simulink model "threephasestator"  (R2016a)
settings: Solver=VariableStepAuto  StartTime=0.0  StopTime=10.0  RelTol=1e-3
undefined symbols (not defined in the file): Lph, Rph
settings Model: Creator=rtw141  LastModifiedBy=rtw141
settings GRTTargetCC: GeneratePreprocessorConditionals=Use local settings

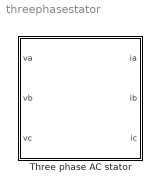
== system threephasestator ==
  Three phase AC stator : Subsystem

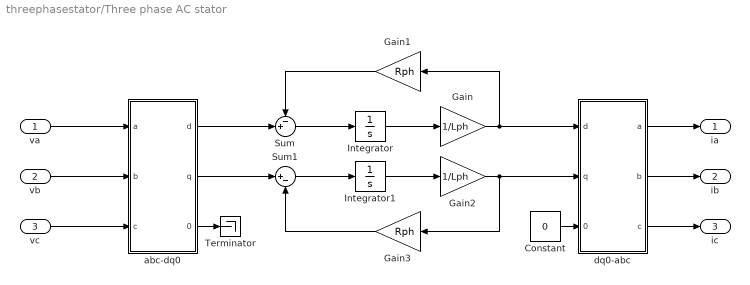
== system threephasestator/Three phase AC stator ==
  va : Inport
  vb : Inport  Port=2
  vc : Inport  Port=3
  Constant : Constant  Value=0
  Gain : Gain  Gain=1/Lph
  Gain1 : Gain  Gain=Rph
  Gain2 : Gain  Gain=1/Lph
  Gain3 : Gain  Gain=Rph
  Integrator : Integrator
  Integrator1 : Integrator
  Sum : Sum  Inputs=-+|
  Sum1 : Sum  Inputs=|+-
  Terminator : Terminator
  abc-dq0 : Subsystem
  dq0-abc : Subsystem
  ia : Outport
  ib : Outport  Port=2
  ic : Outport  Port=3
  wires:
  vc/1 -> abc-dq0/3(c)
  abc-dq0/3(0) -> Terminator/1
  va/1 -> abc-dq0/1(a)
  vb/1 -> abc-dq0/2(b)
  Gain3/1 -> Sum1/2
  Integrator/1 -> Gain/1
  dq0-abc/3(c) -> ic/1
  Sum/1 -> Integrator/1
  Gain2/1 -> dq0-abc/2(q), Gain3/1
  Gain1/1 -> Sum/1
  dq0-abc/1(a) -> ia/1
  abc-dq0/1(d) -> Sum/2
  Sum1/1 -> Integrator1/1
  Integrator1/1 -> Gain2/1
  Gain/1 -> dq0-abc/1(d), Gain1/1
  abc-dq0/2(q) -> Sum1/1
  dq0-abc/2(b) -> ib/1
  Constant/1 -> dq0-abc/3(0)

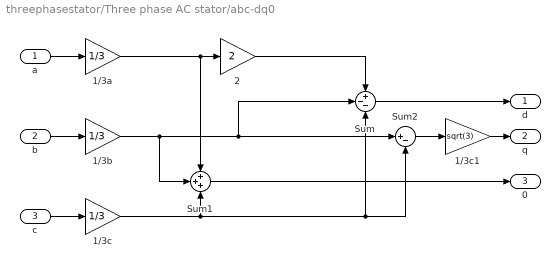
== system threephasestator/Three phase AC stator/abc-dq0 ==
  a : Inport
  b : Inport  Port=2
  c : Inport  Port=3
  1/3a : Gain  Gain=1/3
  1/3b : Gain  Gain=1/3
  1/3c : Gain  Gain=1/3
  1/3c1 : Gain  Gain=sqrt(3)
  2 : Gain  Gain=2
  Sum : Sum  Inputs=+--
  Sum1 : Sum  Inputs=+++
  Sum2 : Sum  Inputs=|+-
  d : Outport
  q : Outport  Port=2
  0 : Outport  Port=3
  wires:
  c/1 -> 1/3c/1
  b/1 -> 1/3b/1
  a/1 -> 1/3a/1
  1/3a/1 -> Sum1/1, 2/1
  2/1 -> Sum/1
  1/3b/1 -> Sum1/2, Sum2/1, Sum/2
  Sum/1 -> d/1
  1/3c/1 -> Sum1/3, Sum2/2, Sum/3
  Sum1/1 -> 0/1
  Sum2/1 -> 1/3c1/1
  1/3c1/1 -> q/1

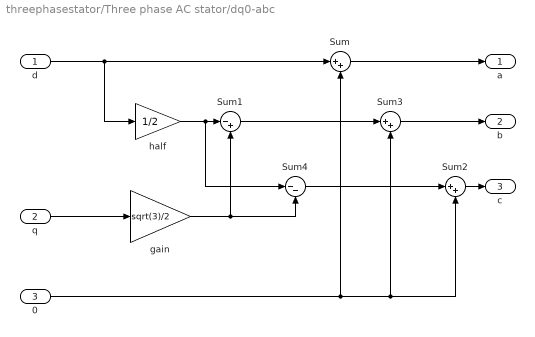
== system threephasestator/Three phase AC stator/dq0-abc ==
  d : Inport
  q : Inport  Port=2
  0 : Inport  Port=3
  Sum : Sum  Inputs=|++
  Sum1 : Sum  Inputs=|-+
  Sum2 : Sum  Inputs=|++
  Sum3 : Sum  Inputs=|++
  Sum4 : Sum  Inputs=|--
  gain : Gain  Gain=sqrt(3)/2
  half : Gain  Gain=1/2
  a : Outport
  b : Outport  Port=2
  c : Outport  Port=3
  wires:
  Sum/1 -> a/1
  d/1 -> half/1, Sum/1
  Sum1/1 -> Sum3/1
  0/1 -> Sum/2, Sum2/2, Sum3/2
  q/1 -> gain/1
  gain/1 -> Sum4/2, Sum1/2
  Sum2/1 -> c/1
  Sum3/1 -> b/1
  half/1 -> Sum4/1, Sum1/1
  Sum4/1 -> Sum2/1
